simulink model "Bi_Directional_DC_DC_converter"  (R2024a)
settings: Solver=VariableStepAuto  StartTime=0.0  StopTime=10.0  RelTol=1e-3
undefined symbols (not defined in the file): Ion, Lithium
libraries: spsSeriesRLCBranchLib x3, spsBatteryLib x2, spsMosfetLib x2, spsVoltageMeasurementLib x2, spsSawtoothGeneratorLib x1, sps_lib x1
settings Model: Creator=RGUKT  LastModifiedBy=RGUKT

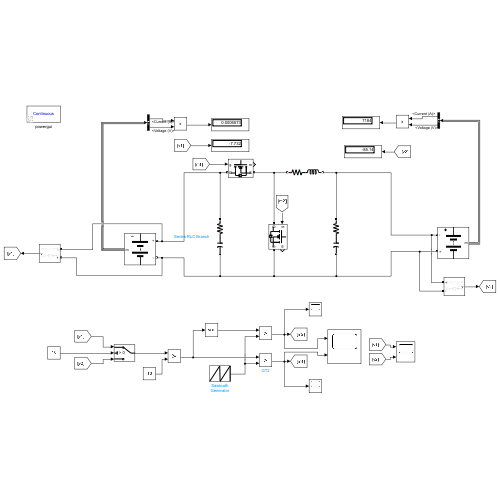
[thumbnail: Simulink's stored preview of the top-level diagram]
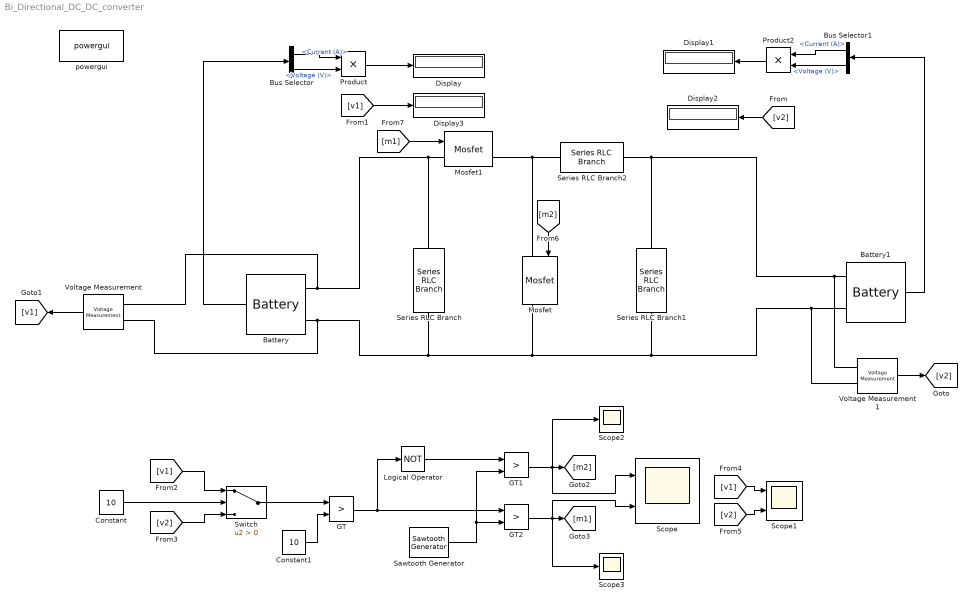
== system Bi_Directional_DC_DC_converter ==
  Battery : spsBatteryLib/Battery  BatType=Lithium-Ion  ShowTempParam=off  ThermalPreset=no  ShowAgeParam=off  NomV=7.2  NomQ=5.4  SOC=100  Batt_Tr=30  PresetModel=on  MaxQ=5.4  MinV=5.4  FullV=8.3807  Dis_rate=2.3478  R=0.013333  Normal_OP=4.8835  expZone="[7.7788      0.2653]"  current=[6.5 13 32.5]  Units=Time  Tci=20  NomT=20  T2=-30  MaxQ2=4.8  FullV2=7.1  Normal_OP2=5.655  expZone2="[6.58           1]"  Rca=0.6  ti=2000  Dp=0  Neq0=0  Tsim=1e6  Ta1=25  Qeol=5.4*0.9  Reol=0.013333*1.2  Char_age=[2.3478, 3]  Dis_age=[2.3478, 10]  N1=1500  N2=10500  N3=1000  N4=1400  Ta2=45  N5=950
  Battery1 : spsBatteryLib/Battery  BatType=Lithium-Ion  ShowTempParam=off  ThermalPreset=no  ShowAgeParam=off  NomV=100  NomQ=5.4  SOC=100  Batt_Tr=30  PresetModel=on  MaxQ=5.4  MinV=75  FullV=116.3987  Dis_rate=2.3478  R=0.18519  Normal_OP=4.8835  expZone="[108.0386     0.2653043]"  current=[6.5 13 32.5]  Units=Time  Tci=20  NomT=20  T2=-30  MaxQ2=4.8  FullV2=7.1  Normal_OP2=5.655  expZone2="[6.58           1]"  Rca=0.6  ti=2000  Dp=0  Neq0=0  Tsim=1e6  Ta1=25  Qeol=5.4*0.9  Reol=0.013333*1.2  Char_age=[2.3478, 3]  Dis_age=[2.3478, 10]  N1=1500  N2=10500  N3=1000  N4=1400  Ta2=45  N5=950
  Bus Selector : BusSelector  OutputSignals=Current (A),Voltage (V)
  Bus Selector1 : BusSelector  OutputSignals=Current (A),Voltage (V)
  Constant : Constant  Value=10
  Constant1 : Constant  Value=10
  Display{,1..3} (4 alike) : Display
  GT : RelationalOperator  Operator=>  OutDataTypeStr=boolean  RndMeth=Simplest  InputSameDT=off
  GT1 : RelationalOperator  Operator=>  OutDataTypeStr=boolean  RndMeth=Simplest  InputSameDT=off
  GT2 : RelationalOperator  Operator=>  OutDataTypeStr=boolean  RndMeth=Simplest  InputSameDT=off
  Logical Operator : Logic  Operator=NOT  AllPortsSameDT=off  OutDataTypeStr=boolean
  Mosfet : spsMosfetLib/Mosfet  Ron=0.1  Lon=0  Rd=0.01  Vfd=0  IC=0  Rs=1e5  Cs=inf  Measurements=on
  Mosfet1 : spsMosfetLib/Mosfet  Ron=0.1  Lon=0  Rd=0.01  Vfd=0  IC=0  Rs=1e5  Cs=inf  Measurements=on
  Product : Product
  Product2 : Product
  Sawtooth Generator : spsSawtoothGeneratorLib/Sawtooth Generator  Freq=50  Phase=0  Ts=0
  Scope : Scope  NumInputPorts=2
  Scope1 : Scope  NumInputPorts=2
  Scope2 : Scope
  Scope3 : Scope
  Series RLC Branch : spsSeriesRLCBranchLib/Series RLC Branch  LConnTagsString=__new0  RConnTagsString=__new0  BranchType=RC  Resistance=1  Inductance=1e-3  SetiL0=off  InitialCurrent=0  Capacitance=1e-6  Setx0=off  InitialVoltage=0  Measurements=None
  Series RLC Branch1 : spsSeriesRLCBranchLib/Series RLC Branch  LConnTagsString=__new0  RConnTagsString=__new0  BranchType=RC  Resistance=1  Inductance=1e-3  SetiL0=off  InitialCurrent=0  Capacitance=1e-6  Setx0=off  InitialVoltage=0  Measurements=None
  Series RLC Branch2 : spsSeriesRLCBranchLib/Series RLC Branch  LConnTagsString=__new0  RConnTagsString=__new0  BranchType=RL  Resistance=1  Inductance=1e-3  SetiL0=off  InitialCurrent=0  Capacitance=1e-6  Setx0=off  InitialVoltage=0  Measurements=None
  Switch : Switch  Criteria=u2 > Threshold  SaturateOnIntegerOverflow=off  InputSameDT=off
  Voltage Measurement : spsVoltageMeasurementLib/Voltage Measurement  PhasorSimulation=off  OutputType=Complex  PSBequivalent=0
  Voltage Measurement1 : spsVoltageMeasurementLib/Voltage Measurement  PhasorSimulation=off  OutputType=Complex  PSBequivalent=0
  powergui : sps_lib/powergui  Priority=1  SimulationMode=Continuous  SampleTime=10  frequency=60  Iterations=50  frequencyindice=0  Pbase=100e6  ErrMax=1e-4  UnitsV=kV  UnitsW=MW  buscounter=0  FunctionMessages=off  echomessages=off  EnableUseOfTLC=off  CurrentSourceSwitches=off  DisableSnubberDevices=off  DisableRonSwitches=off  DisableVfSwitches=off  DisplayEquations=off  AutomaticDiscreteSolvers=off  SolverType=Tustin/Backward Euler (TBE)  Interpol=off  ExternalGateDelay=off  methode=off  Ts=100  x0status=blocks  SPID=on  SwTol=0  HookPort=off  NonlinearTolerance=1e-4  nMaxIteration=100  ContinueOnMaxIteration=off  RestoreLinks=warning  ResistiveCurrentMeasurement=off  Frange=[0:2:500]  Ylog=off  Xlog=on  ShowGrid=off  save=off  variable=ZData  structure=0  ZoomFFT=off  StartTime=0.0  cycles=1  DisplayStyle=1  fundamental=60  FreqAxis=off  MaxFrequency=1000  frequencyindicesteady=1  RmsSteady=1  display=off
  wires:
  Battery/1 -> Bus Selector/1
  Bus Selector/1 -> Product/1  "<Current (A)>"
  Bus Selector/2 -> Product/2  "<Voltage (V)>"
  Product/1 -> Display/1
  Bus Selector1/1 -> Product2/1  "<Current (A)>"
  Bus Selector1/2 -> Product2/2  "<Voltage (V)>"
  Battery1/1 -> Bus Selector1/1
  Product2/1 -> Display1/1
  Voltage Measurement1/1 -> [v2]
  Voltage Measurement/1 -> [v1]
  [v2] -> Display2/1
  [v1] -> Display3/1
  [v1] -> Switch/1
  [v2] -> Switch/3
  Constant/1 -> Switch/2
  Switch/1 -> GT/1
  Constant1/1 -> GT/2
  GT/1 -> GT2/1, Logical Operator/1
  Logical Operator/1 -> GT1/1
  Sawtooth Generator/1 -> GT1/2, GT2/2
  GT1/1 -> Scope/1, [m2], Scope2/1
  GT2/1 -> Scope/2, [m1], Scope3/1
  [v1] -> Scope1/1
  [v2] -> Scope1/2
  [m2] -> Mosfet/1
  [m1] -> Mosfet1/1
  connections:
  Battery/LConn1 -- Voltage Measurement/LConn2 -- Series RLC Branch/LConn1 -- Mosfet1/LConn1
  Battery/LConn2 -- Voltage Measurement/LConn1 -- Voltage Measurement1/LConn2 -- Battery1/LConn1 -- Series RLC Branch1/RConn1 -- Mosfet/RConn1 -- Series RLC Branch/RConn1
  Series RLC Branch1/LConn1 -- Series RLC Branch2/RConn1 -- Voltage Measurement1/LConn1 -- Battery1/LConn2
  Mosfet/LConn1 -- Series RLC Branch2/LConn1 -- Mosfet1/RConn1
